simulink model "ex1"  (Simulink 6.0)
settings: Solver=ode45  StartTime=0.0  StopTime=10.0  RelTol=1e-3
settings Model: LastModifiedBy=student

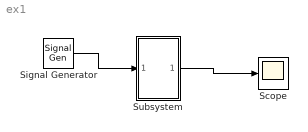
== system ex1 ==
  Scope : Scope
  Signal Generator : SignalGenerator
  Subsystem : Subsystem  mask{a=0.1}
      mask prompts: a "factorul de amplificare"
      mask Display: image(imread('b747.jpg'))
  wires:
  Signal Generator/1 -> Subsystem/1(In1)
  Subsystem/1(Out1) -> Scope/1

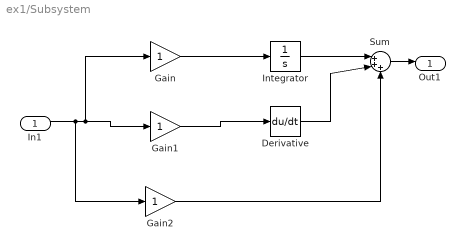
== system ex1/Subsystem ==
  In1 : Inport  Port=1  LatchInput=off
  Derivative : Derivative
  Gain : Gain
  Gain1 : Gain
  Gain2 : Gain
  Integrator : Integrator  InitialCondition=a
  Sum : Sum  Inputs=|+++
  Out1 : Outport
  wires:
  Gain/1 -> Integrator/1
  Integrator/1 -> Sum/1
  Gain1/1 -> Derivative/1
  Derivative/1 -> Sum/2
  Gain2/1 -> Sum/3
  In1/1 -> Gain1/1, Gain/1, Gain2/1
  Sum/1 -> Out1/1
